simulink model "INV_test"  (R2016b)
settings: Solver=FixedStepAuto  StartTime=0.0  StopTime=2  FixedStep=0.02  RelTol=1e-3
values from neighbouring files (symbols this model uses):
  inverter_eff = 0.93    [Init_PI_reg.m]    (also in Initial_test.m; battery_test_res.mat; body_test_res.mat; motor_test_res.mat)
  U_uvp = 330    [Init_PI_reg.m]    (also in Initial_test.m; battery_test_res.mat; body_test_res.mat; motor_test_res.mat)
settings Model: Creator=a037702  LastModifiedBy=a037702

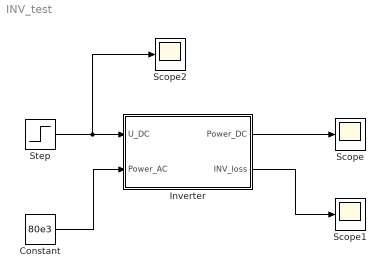
== system INV_test ==
  Constant : Constant  Value=80e3
  Inverter : Subsystem
  Scope : Scope
  Scope1 : Scope
  Scope2 : Scope
  Step : Step  Before=400  After=300  SampleTime=0
  wires:
  Step/1 -> Inverter/1(U_DC), Scope2/1
  Constant/1 -> Inverter/2(Power_AC)
  Inverter/1(Power_DC) -> Scope/1
  Inverter/2(INV_loss) -> Scope1/1

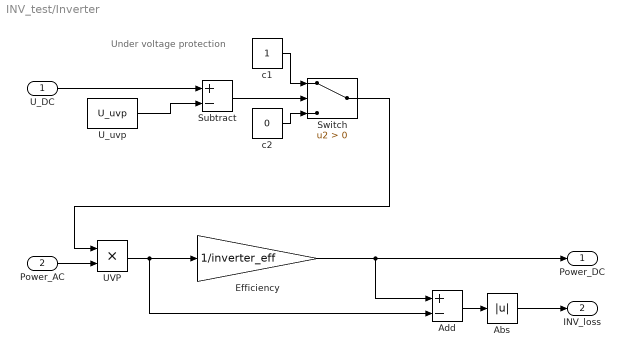
== system INV_test/Inverter ==
  note: Under voltage protection
  U_DC : Inport
  Power_AC : Inport  Port=2
  Abs : Abs
  Add : Sum  Inputs=+-
  Efficiency : Gain  Gain=1/inverter_eff
  Subtract : Sum  Inputs=+-
  Switch : Switch  Criteria=u2 > Threshold
  UVP : Product
  U_uvp : Constant  Value=U_uvp
  c1 : Constant
  c2 : Constant  Value=0
  Power_DC : Outport
  INV_loss : Outport  Port=2
  wires:
  UVP/1 -> Efficiency/1, Add/2
  Add/1 -> Abs/1
  U_uvp/1 -> Subtract/2
  U_DC/1 -> Subtract/1
  Subtract/1 -> Switch/2
  Efficiency/1 -> Power_DC/1, Add/1
  Switch/1 -> UVP/1
  c1/1 -> Switch/1
  c2/1 -> Switch/3
  Power_AC/1 -> UVP/2
  Abs/1 -> INV_loss/1
